simulink model "PIDcontrol"  (Simulink 8.5)
settings: Solver=ode45  StartTime=0.0  StopTime=2500  RelTol=1e-3
libraries: simulink x1
settings Model: Creator=YH  LastModifiedBy=YH
settings DataIOCC: SignalLoggingSaveFormat=Dataset
settings OptimizationCC: ExpressionDepthLimit=128
settings DebuggingCC: UnderspecifiedInitializationDetection=Simplified  MergeDetectMultiDrivingBlocksExec=error  FcnCallInpInsideContextMsg=EnableAllAsError  StateNameClashWarn=none
settings GRTTargetCC: CombineOutputUpdateFcns=on  GRTInterface=off

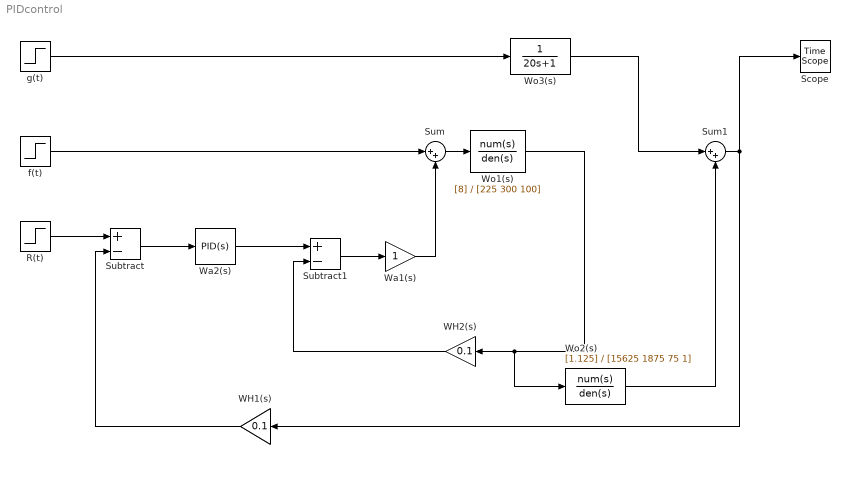
== system PIDcontrol ==
  R(t) : Step  SampleTime=0
  Scope : TimeScope
  Subtract : Sum  Inputs=+-
  Subtract1 : Sum  Inputs=+-
  Sum : Sum  Inputs=|++
  Sum1 : Sum  Inputs=|++
  WH1(s) : Gain  Gain=0.1
  WH2(s) : Gain  Gain=0.1
  Wa1(s) : Gain
  Wa2(s) : simulink/Continuous/PID Controller  Controller=PID  TimeDomain=Continuous-time  SampleTime=-1  IntegratorMethod=Forward Euler  FilterMethod=Forward Euler  Form=Parallel  UseFilter=on  ControllerParametersSource=internal  P=1  I=2  D=1  N=100  InitialConditionSource=internal  InitialConditionForIntegrator=0  InitialConditionForFilter=0  ExternalReset=none  LimitOutput=off  UpperSaturationLimit=inf  LowerSaturationLimit=-inf  LinearizeAsGain=on  AntiWindupMode=none  Kb=1  TrackingMode=off  Kt=1  PParamMin=[]  PParamMax=[]  IParamMin=[]  IParamMax=[]  DParamMin=[]  DParamMax=[]  NParamMin=[]  NParamMax=[]  KbParamMin=[]  KbParamMax=[]  KtParamMin=[]  KtParamMax=[]  POutMin=[]  POutMax=[]  IOutMin=[]  IOutMax=[]  DOutMin=[]  DOutMax=[]  NOutMin=[]  NOutMax=[]  KbOutMin=[]  KbOutMax=[]  KtOutMin=[]  KtOutMax=[]  IntegratorOutMin=[]  IntegratorOutMax=[]  FilterOutMin=[]  FilterOutMax=[]  SumOutMin=[]  SumOutMax=[]  SumI1OutMin=[]  SumI1OutMax=[]  SumI2OutMin=[]  SumI2OutMax=[]  SumI3OutMin=[]  SumI3OutMax=[]  SumDOutMin=[]  SumDOutMax=[]  SaturationOutMin=[]  SaturationOutMax=[]  IntegratorContinuousStateAttributes=''  IntegratorStateMustResolveToSignalObject=off  IntegratorRTWStateStorageClass=Auto  FilterContinuousStateAttributes=''  FilterStateMustResolveToSignalObject=off  FilterRTWStateStorageClass=Auto  DifferentiatorICPrevScaledInput=0  DifferentiatorOutMin=[]  DifferentiatorOutMax=[]
  Wo1(s) : TransferFcn  Numerator=[8]  Denominator=[225 300 100]
  Wo2(s) : TransferFcn  Numerator=[1.125]  Denominator=[15625 1875 75 1]
  Wo3(s) : TransferFcn  Denominator=[20 1]
  f(t) : Step  SampleTime=0
  g(t) : Step  SampleTime=0
  wires:
  R(t)/1 -> Subtract/1
  WH1(s)/1 -> Subtract/2
  Sum1/1 -> Scope/1, WH1(s)/1
  g(t)/1 -> Wo3(s)/1
  Wo3(s)/1 -> Sum1/1
  Wo1(s)/1 -> Wo2(s)/1, WH2(s)/1
  Wo2(s)/1 -> Sum1/2
  Sum/1 -> Wo1(s)/1
  f(t)/1 -> Sum/1
  Wa1(s)/1 -> Sum/2
  Wa2(s)/1 -> Subtract1/1
  Subtract1/1 -> Wa1(s)/1
  Subtract/1 -> Wa2(s)/1
  WH2(s)/1 -> Subtract1/2
